simulink model "PlanarChassisVehicleModel"  (R2021a)
settings: Solver=VariableStepAuto  StartTime=0.0  StopTime=10.0  RelTol=1e-3
(part 1 of 2)
settings Model: Creator=jpchi  LastModifiedBy=jpchi

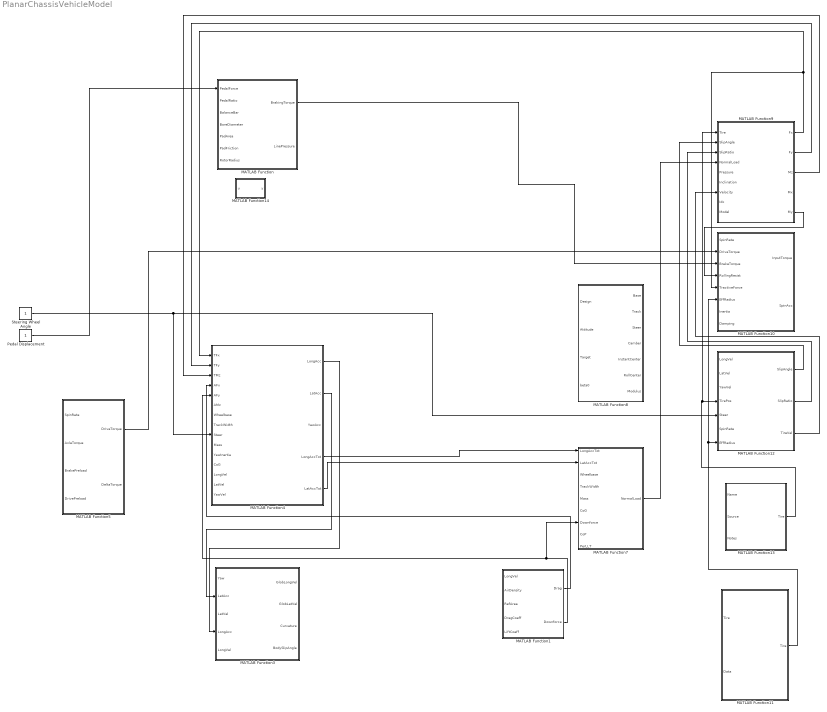
== system PlanarChassisVehicleModel ==
  MATLAB Function : MATLAB Function  TreatAsAtomicUnit=on
  MATLAB Function1 : MATLAB Function  TreatAsAtomicUnit=on
  MATLAB Function10 : MATLAB Function  TreatAsAtomicUnit=on
  MATLAB Function11 : MATLAB Function  TreatAsAtomicUnit=on
  MATLAB Function12 : MATLAB Function  TreatAsAtomicUnit=on
  MATLAB Function13 : MATLAB Function  TreatAsAtomicUnit=on
  MATLAB Function14 : MATLAB Function  TreatAsAtomicUnit=on
  MATLAB Function3 : MATLAB Function  TreatAsAtomicUnit=on
  MATLAB Function4 : MATLAB Function  TreatAsAtomicUnit=on
  MATLAB Function5 : MATLAB Function  TreatAsAtomicUnit=on
  MATLAB Function7 : MATLAB Function  TreatAsAtomicUnit=on
  MATLAB Function8 : MATLAB Function  TreatAsAtomicUnit=on
  MATLAB Function9 : MATLAB Function  TreatAsAtomicUnit=on
  Pedal Displacement : Constant
  Steering Wheel Angle : Constant
  wires:
  Pedal Displacement/1 -> MATLAB Function/1(PedalForce)
  MATLAB Function12/1(SlipAngle) -> MATLAB Function9/2(SlipAngle)
  MATLAB Function12/2(SlipRatio) -> MATLAB Function9/3(SlipRatio)
  MATLAB Function/1(BrakingTorque) -> MATLAB Function10/3(BrakeTorque)
  Steering Wheel Angle/1 -> MATLAB Function4/9(Steer), MATLAB Function12/5(Steer)
  MATLAB Function9/1(Fx) -> MATLAB Function4/1(TFx), MATLAB Function10/5(TractiveForce)
  MATLAB Function9/2(Fy) -> MATLAB Function4/2(TFy)
  MATLAB Function9/3(Mz) -> MATLAB Function4/3(TMz)
  MATLAB Function9/5(My) -> MATLAB Function10/4(RollingResist)
  MATLAB Function12/3(TireVel) -> MATLAB Function9/7(Velocity)
  MATLAB Function4/1(LongAcc) -> MATLAB Function3/4(LongAcc)
  MATLAB Function4/2(LatAcc) -> MATLAB Function3/2(LatAcc)
  MATLAB Function5/1(DriveTorque) -> MATLAB Function10/2(DriveTorque)
  MATLAB Function11/1(Tire) -> MATLAB Function12/7(EffRadius), MATLAB Function10/6(EffRadius)
  MATLAB Function13/1(Tire) -> MATLAB Function9/1(Tire), MATLAB Function12/4(TirePos)
  MATLAB Function1/1(Drag) -> MATLAB Function4/4(AFx)
  MATLAB Function1/2(Downforce) -> MATLAB Function7/7(Downforce), MATLAB Function4/5(AFy)
  MATLAB Function4/4(LongAccTot) -> MATLAB Function7/1(LongAccTot)
  MATLAB Function4/5(LatAccTot) -> MATLAB Function7/2(LatAccTot)
  MATLAB Function7/1(NormalLoad) -> MATLAB Function9/4(NormalLoad)

== matlab function PlanarChassisVehicleModel/MATLAB Function7 ==
  data: LongAccTot input; NormalLoad output; LatAccTot input; Wheelbase input; TrackWidth input; Mass input; CoG input; Downforce input; CoP input; PerLLT input
function NormalLoad  = SimplifiedWeightTransfer( LongAccTot, LatAccTot, ...
        Wheelbase, TrackWidth, Mass, CoG, Downforce, CoP, PerLLT ) 
%% SimplifiedWeightTransfer - Simplified Normal Loads
% Computes tire normal loads using simplified weight transfer and
% aerodynamic loading.
% 
% Inputs:
%   LongAccTot - (n,1 numeric) Total Longitudinal Acceleration     {a_x}   [m/s^2]
%   LatAccTot  - (n,1 numeric) Total Lateral Acceleration          {a_y}   [m/s^2]
%   Wheelbase  - (n,1 numeric) Wheelbase                           {L}     [m]
%   TrackWidth - (n,2 numeric) Track Width                         {t_w}   [m]
%   Mass       - (n,1 numeric) Total Vehicle Mass                  {m}     [kg]
%   CoG        - (n,3 numeric) Center of Gravity                   {CoG}   [m]
%   Downforce  - (n,1 numeric) Aerodynamic Downforce               {A_F_z} [N]
%   CoP        - (n,3 numeric) Center of Pressure                  {CoP}   [m]
%   PerLLT     - (n,1 numeric) Percent Front Lateral Load Transfer {%_LLT} [ ]
%
% Outputs:
%   NormalLoad - (n,4 numeric) Tire Normal Loads                   {T_F_z} [N]
%
% Notes:
%
% Author(s): 
% Blake Christierson (bechristierson@ucdavis.edu) [Sep 2018 - Jun 2021] 
% 
% Last Updated: 30-May-2021

%% Test Case
if nargin == 0
    LongAccTot = -0.5 .* 9.81;
    LatAccTot  =  0.7 .* 9.81;
    
    Wheelbase = 1.575;
    TrackWidth = [1.22, 1.23];
    
    Mass = 275;
    CoG  = [(0.47-0.5)*Wheelbase, 0, 0.25];
    
    Downforce = 200;
    CoP  = [(0.4-0.5)*Wheelbase, 0, 0];
    
    PerLLT = 0.6;
    
    [NormalLoad] = SimplifiedWeightTransfer( LongAccTot, LatAccTot, ...
        Wheelbase, TrackWidth, Mass, CoG, Downforce, CoP, PerLLT ) %#ok<NOPRT>
    
    return
end

%% Computation
NormalLoad = zeros( [size( LongAccTot ), 4] );

%%% Total Weight Transfer
dFzx = Mass .* LongAccTot .* CoG(:,3) ./ Wheelbase;
dFzy = Mass .* LatAccTot  .* CoG(:,3) ./ mean(TrackWidth, 2);

%%% Static Wheel Loads
MassBal = (CoG(:,1) + Wheelbase./2) ./ Wheelbase;
AeroBal = (CoP(:,1) + Wheelbase./2) ./ Wheelbase;

NormalLoad(:,1:2) = (MassBal .* Mass .* 9.81 + AeroBal .* Downforce) / 2;
NormalLoad(:,3:4) = ((1-MassBal) .* Mass .* 9.81 + (1-AeroBal) .* Downforce) / 2;

%%% Dynamic Wheel Loads
NormalLoad(:,1) = NormalLoad(:,1) + (-0.5.*dFzx - PerLLT    .*dFzy)/2;
NormalLoad(:,2) = NormalLoad(:,2) + (-0.5.*dFzx + PerLLT    .*dFzy)/2;
NormalLoad(:,3) = NormalLoad(:,3) + ( 0.5.*dFzx - (1-PerLLT).*dFzy)/2;
NormalLoad(:,4) = NormalLoad(:,4) + ( 0.5.*dFzx + (1-PerLLT).*dFzy)/2;

end

== matlab function PlanarChassisVehicleModel/MATLAB Function8 ==
  data: Design input; Base output; Attitude input; Target input; beta0 input; Track output; Steer output; Camber output; InstantCenter output; RollCenter output; Modulus output
function [Base, Track, Steer, Camber, InstantCenter, RollCenter, Modulus] = ...
    KinematicsEvaluation( Design, Attitude, Target, beta0 )
%% Define Coordinate Transformations
if strcmp(Target.Axle, 'Front')
    L = Target.Wheelbase;
else
    L = -Target.Wheelbase;
end

RotX = @(t) [1       0       0      ;  0       cosd(t) sind(t);  0       -sind(t) cosd(t)];
RotY = @(t) [cosd(t) 0       sind(t);  0       1       0      ; -sind(t)  0       cosd(t)];
RotZ = @(t) [cosd(t) sind(t) 0      ; -sind(t) cosd(t) 0      ;  0        0       1      ];

% bTw = @(pW,phi,theta) RotX(phi)    * RotY(theta) * (pW - Target.CG' - [L/2 0 0]'); %world to body
wTb = @(pB,phi,theta) RotY(theta)' * RotX(phi)'  *  pB + Target.CG' + [-L/2 0 Attitude.Ride-50.8]'; %body to world


% tTw = @(pW,xT,yT,gamma,phi,delta) RotZ(delta) * RotX(gamma)  * RotY(phi) * (pW - [xT yT Target.Rl]'); %world to tire
% wTt = @(pT,xT,yT,gamma,phi,delta) RotY(phi)'  * RotX(gamma)' * RotZ(delta)' *  pT + [xT yT Target.Rl]' ; %old copy - tire to world
% wTt = @(pT,xT,yT,gamma,delta) RotX(gamma)' * RotZ(delta)' *  pT + [xT yT 0]' ; %tire to world
    
% bTw = @(pW,phi,theta) RotX(phi)    * RotY(theta) * (pW - Target.CG' - [L/2 0 0]');
wTb = @(pB,phi,theta) RotY(theta)' * RotX(phi)'  *  pB + Target.CG' + [-L/2 0 Attitude.Ride-50.8]';

%tTw = @(pW,xT,yT,gamma,phi,delta) RotZ(delta) * RotX(gamma)  * RotY(phi) * (pW - [xT yT Target.Rl]');
% wTt = @(pT,xT,yT,gamma,phi,delta) RotY(phi)'  * RotX(gamma)' * RotZ(delta)' *  pT + [xT yT Target.Rl]' ;

% whTt = @
tTwh = @(pWH,camber,KPI,caster) RotY(caster)' * RotX(KPI)' * ( ( RotX(-camber)' * pWH ) + [0 Target.Scrub 0]' ) + [0 0 Target.Rl/cosd(KPI)]';
% tbTwh = @ (pWH) pWH - Design.tr;

% laTb = @(pB,beta) RotX(beta)            * RotZ(Design.a.LA(2))  * RotY(Design.a.LA(1)) * (pB - (Design.p.LAb + [L/2 0 Target.Ride-Target.CG(3)]')); %body to lower a-arm
bTla = @(pA,beta) RotY(Design.a.LA(1))' * RotZ(Design.a.LA(2))' * RotX(beta)'          *  pA +  Design.p.LAb + [L/2 0 Target.Ride-Target.CG(3)]'  ; %lower a-arm to body

% uaTb = @(pB,beta) RotX(beta)            * RotZ(Design.a.UA(2))  * RotY(Design.a.UA(1)) * (pB - (Design.p.UAb + [L/2 0 Target.Ride-Target.CG(3)]')); %body to upper a-arm
bTua = @(pA,beta) RotY(Design.a.UA(1))' * RotZ(Design.a.UA(2))' * RotX(beta)'          *  pA +  Design.p.UAb + [L/2 0 Target.Ride-Target.CG(3)]'  ; %upper a-arm to body

% lbTla = @(pA ,beta1,beta2,beta3) RotZ(beta3)  * RotX(beta1)  * RotY(beta2)  * (pA  - [0 Design.L.LA 0]'); %lower a-arm to lower ball joint
laTlb = @(pLB,beta1,beta2,beta3) RotY(beta2)' * RotX(beta1)' * RotZ(beta3)' *  pLB + [0 Design.L.LA 0]' ; %lower ball joint to lower a-arm

lbTt = @(pT ) pT  - Design.p.LBt; %tire to lower ball joint
% tTlb = @(pLB) pLB + Design.p.LBt; %lower ball joint to tire

% trTb = @(pB ,beta1,beta2) RotZ(beta2)  * RotX(beta1)  * (pB  - (Design.p.TAb + [L/2 Attitude.Steer Target.Ride-Target.CG(3)]')); %body to tie rod
bTtr = @(pTR,beta1,beta2) RotX(beta1)' * RotZ(beta2)' *  pTR +  Design.p.TAb + [L/2 Attitude.Steer Target.Ride-Target.CG(3)]'  ; %tie rod to body

% laTb = @(pB,beta) RotX(beta)            * RotZ(Design.a.LA(2))  * RotY(Design.a.LA(1)) * (pB - (Design.p.LAb + [L/2 0 Target.Ride-Target.CG(3)]'));
bTla = @(pA,beta) RotY(Design.a.LA(1))' * RotZ(Design.a.LA(2))' * RotX(beta)'          *  pA +  Design.p.LAb + [L/2 0 Target.Ride-Target.CG(3)]'  ; 

% uaTb = @(pB,beta) RotX(beta)            * RotZ(Design.a.UA(2))  * RotY(Design.a.UA(1)) * (pB - (Design.p.UAb + [L/2 0 Target.Ride-Target.CG(3)]')); 
bTua = @(pA,beta) RotY(Design.a.UA(1))' * RotZ(Design.a.UA(2))' * RotX(beta)'          *  pA +  Design.p.UAb + [L/2 0 Target.Ride-Target.CG(3)]'  ;

% lbTla = @(pA ,beta1,beta2,beta3) RotZ(beta3)  * RotX(beta1)  * RotY(beta2)  * (pA  - [0 Design.L.LA 0]'); 
laTlb = @(pLB,beta1,beta2,beta3) RotY(beta2)' * RotX(beta1)' * RotZ(beta3)' *  pLB + [0 Design.L.LA 0]' ; 

lbTt = @(pT ) pT  - Design.p.LBt; 
% tTlb = @(pLB) pLB + Design.p.LBt; 

% trTb = @(pB ,beta1,beta2) RotZ(beta2)  * RotX(beta1)  * (pB  - (Design.p.TAb + [L/2 Attitude.Steer Target.Ride-Target.CG(3)]')); 
bTtr = @(pTR,beta1,beta2) RotX(beta1)' * RotZ(beta2)' *  pTR +  Design.p.TAb + [L/2 Attitude.Steer Target.Ride-Target.CG(3)]'  ;

%% Optimization Problem Setup & Execution
if nargin < 4
    beta0 = [ 1, ... % Lower A-Arm Rotation
              5, ... % Upper A-Arm Rotation
              0, 0, ... % Tie Rod (x,z)-Axis Rotations
              0, 0, 0]; % Lower Ball Joint (x,y,z)-Axis Rotations
end

lb = [-10 -20 -20 -30 -10 -10 -40];
ub = [ 30  35  30  30  10  10  40];

ObjFun = @(beta) ObjectiveFunction( beta, Design, Attitude, Target );
[beta, fval] = fmincon( ObjFun, beta0, [], [], [], [], lb, ub, [], optimset( 'Display', 'off' ) );

[Base, Track, Steer, Camber, InstantCenter, RollCenter, Modulus] = ...
    SuspensionMetrics( beta, Attitude, Target );

%%% Local Functions
    function Fval = ObjectiveFunction( beta, Design, Attitude, Target )
        UB = bTla( laTlb( lbTt(Design.p.UBt), beta(5), beta(6), beta(7) ), beta(1) ) - ...
             bTua( [0 Design.L.UA 0]', beta(2) );
        
        TB = bTla( laTlb( lbTt(Design.p.TBt), beta(5), beta(6), beta(7) ), beta(1) ) - ...
             bTtr( [0 Design.L.TR 0]', beta(3), beta(4) );
        
        oT = wTb( bTla( laTlb( -Design.p.LBt, beta(5), beta(6), beta(7) ), beta(1) ), Attitude.Roll, Attitude.Pitch );
         
        Rl = oT(3) - Target.Rl;
        
        Fval = norm(UB) + norm(TB) + Rl.^2;
    end

    function [Base, Track, Steer, Camber, InstantCenter, RollCenter, Modulus] = ...
            SuspensionMetrics( beta, Attitude, Target )       
        %%% Wheel Position & Orientation
        % Wheel Position
        T = wTb( bTla( laTlb( lbTt([0 0 0]'), beta(5), beta(6), beta(7) ), beta(1) ), Attitude.Roll, Attitude.Pitch );
        % T = wTt([0 0 0]', Steer, Camber)
        Base = T(1);
        Track = T(2);
         
        % Solve for Tire Unit Vectors
        xT = wTb( bTla( laTlb( lbTt([1 0 0]'), beta(5), beta(6), beta(7) ), beta(1) ), Attitude.Roll, Attitude.Pitch );
        % xT = wTt([1 0 0]', Steer, Camber)
        yT = wTb( bTla( laTlb( lbTt([0 1 0]'), beta(5), beta(6), beta(7) ), beta(1) ), Attitude.Roll, Attitude.Pitch );
        % yT = wTt([0 1 0]', Steer, Camber)
        zT = wTb( bTla( laTlb( lbTt([0 0 1]'), beta(5), beta(6), beta(7) ), beta(1) ), Attitude.Roll, Attitude.Pitch );
        % zT = wTt([0 0 1]', Steer, Camber)
        
        xT = xT - T;
        yT = yT - T;
        zT = zT - T;
         
        % Solve for Tire Positions
        posT = wTb( bTla( laTlb( lbTt( tTwh([0 0 0]', Target.Camber, Target.KPI, Target.Caster) ), beta(5), beta(6), beta(7) ),...
            beta(1) ), Attitude.Roll, Attitude.Pitch );
        
        % Solve for Steer & Camber [Sign Issues]
        Camber = acosd( dot( yT, [0 0 1]' ) ) - 90; % Camber Angle [deg]

        k = cross( zT, [0 0 1]' ) ./ sind(Camber); % Camber Rotation Vector
        
        yTa = yT*cosd(Camber) + cross(k,yT)*sind(Camber) + ...
            k*dot(k,yT)*(1-cosd(Camber)); % Ground Parallel Longitudinal Tire Axis
        yTa = yTa ./ norm(yTa);
        
        Steer = -sign(yTa(1)) * acosd( dot( yTa, [0 1 0]' ) ); % Steer Angle [deg]
        
        %%% Roll Geometry Metrics
        pLA = wTb( bTla( [0 0 0]', beta(1) ), Attitude.Roll, Attitude.Pitch );
        pUA = wTb( bTua( [0 0 0]', beta(2) ), Attitude.Roll, Attitude.Pitch );
        pTA = wTb( bTtr( [0 0 0]', beta(3), beta(4) ), Attitude.Roll, Attitude.Pitch );
        
        pLB = wTb( bTla( [0 Design.L.LA 0]', beta(1) ), Attitude.Roll, Attitude.Pitch );
        pUB = wTb( bTua( [0 Design.L.UA 0]', beta(2) ), Attitude.Roll, Attitude.Pitch );
        pTB = wTb( bTtr( [0 Design.L.TR 0]', beta(3), beta(4) ), Attitude.Roll, Attitude.Pitch );
               
        InstantCenter = LineIntersection( pLA(2:3), pLB(2:3), pUA(2:3), pUB(2:3) );
        RollCenter = LineIntersection( InstantCenter, [Track,0], [0,0], [0,1] );
        
        %%% KPI / Scrub Calculator
        
        %%% Steering Effort
%         % Solve for Tire Forces
%         Tire = Target.TireParameter.Tire.Pacejka;
%         SlipAngle   = Steer;         %[degrees]
%         SlipRatio   = 0.00;             %[ ] Assume no slip
%         NormalLoad  = 270 * 9.81/4;  %[N] About 1/4 the weight of the car
%         Pressure    = 70;            %[kPa] 10 psi
%         Inclination = Target.Camber; %[degrees]
%         Velocity    = 10;            %[m/s]
%         Idx         = 1;             %[ ]
%         Model       = struct( 'Pure', 'Pacejka', 'Combined', 'MNC' );
%         
%         [Fx, Fy, Mz, ~, ~] = ContactPatchLoads( Tire, SlipAngle, ...
%             SlipRatio, NormalLoad, Pressure, Inclination, Velocity, Idx, Model );
%         
%         % Solve for Moments from tire and tie rod
%         ToeBase = T-pTB; %distance from tie rod pickup point to center of wheel
%         disT = posT - T; %posT is contact patch, T is center of wheel
%         dirTR = ( pTB-pTA ) ./ ( norm( pTB-pTA ) ); %direction of the force in the tie rod
%         
%         %Solve for Modulus
%         TireForce = [Fx, Fy, Mz]; %tire forces matrix from tire model
%         TireDirection = [ xT; yT ]; %tire direction matrix
%         Modulus = zeros( size(TireForce) ); %initiailize modulus matrix
%         
%         for i = size(TireForce)
%             if i <= size(TireDirection,1)
%                 ModulusMoment = cross( disT, TireDirection(i,:) ); %Tire Moment
%             else
%                 ModulusMoment = [ 0, 0, 1 ]; %Tire Moment
%             end
%             Modulus(i) = [0, 0, ModulusMoment(3)] ./ (cross( ToeBase, dirTR) );
%         end
%         
%         %Solve for Steering Effort
%         TieRodForce = TireForce.*Modulus'; %Solves force into the tie rod
%         SteeringEffort = TieRodForce(2)*( 0.08788 / ( 2*pi ) ); %torque at the steering wheel needed to turn wheel [N*m] (rack travel 87.88mm/deg)
        Modulus = 0;
        
        %%% Debugging
        %{ 
        plot3( LA(1), LA(2), LA(3), 'bx', ...
               UA(1), UA(2), UA(3), 'rx', ...
               TA(1), TA(2), TA(3), 'gx', ...
               LB(1), LB(2), LB(3), 'b+', ...
               UB(1), UB(2), UB(3), 'r+', ...
               TB(1), TB(2), TB(3), 'g+', ...
                T(1),  T(2),  T(3), 'mx');
        quiver3( 0, 0, 0, yT(1), yT(2), yT(3) ); hold on;
        %}
    end

    function pX = LineIntersection(p1, p2, p3, p4)
        pX(1) = det( [det( [p1(1) p1(2); p2(1) p2(2)] ), det( [p1(1) 1; p2(1) 1] ); ...
                      det( [p3(1) p3(2); p4(1) p4(2)] ), det( [p3(1) 1; p4(1) 1] )] ) ./ ...
                det( [det( [p1(1) 1    ; p2(1) 1    ] ), det( [p1(2) 1; p2(2) 1] ); ...
                      det( [p3(1) 1    ; p4(1) 1    ] ), det( [p3(2) 1; p4(2) 1] )] ); 
                  
        pX(2) = det( [det( [p1(1) p1(2); p2(1) p2(2)] ), det( [p1(2) 1; p2(2) 1] ); ...
                      det( [p3(1) p3(2); p4(1) p4(2)] ), det( [p3(2) 1; p4(2) 1] )] ) ./ ...
                det( [det( [p1(1) 1    ; p2(1) 1    ] ), det( [p1(2) 1; p2(2) 1] ); ...
                      det( [p3(1) 1    ; p4(1) 1    ] ), det( [p3(2) 1; p4(2) 1] )] );
    end
end

== matlab function PlanarChassisVehicleModel/MATLAB Function9 ==
  data: Tire input; Fx output; SlipAngle input; SlipRatio input; NormalLoad input; Pressure input; Inclination input; Velocity input; Idx input; Model input; Fy output; Mz output; Mx output; My output
function [Fx, Fy, Mz, Mx, My] = ContactPatchLoads( Tire, ...
    SlipAngle, SlipRatio, ...
    NormalLoad, Pressure, Inclination, Velocity, ...
    Idx, Model )
%% ContactPatchLoads - Tire Load Evaluation
% This script evaluates a Pacejka contact patch tire model using the
% formatted by TireModelFittingMain(). 
% 
% Inputs:
%   Tire          - (struct)      Pacejka Parameters
%   SlipAngle     - (n,1 numeric) Slip Angle          {alpha} [deg]
%   SlipRatio     - (n,1 numeric) Slip Ratio          {kappa} [ ]
%   NormalLoad    - (n,1 numeric) Normal Load         {F_z}   [N]
%   Pressure      - (n,1 numeric) Inflation Pressure  {P_i}   [kPa]
%   Inclination   - (n,1 numeric) Inclination Angle   {gamma} [deg]
%   Velocity      - (n,1 numeric) Center Velocity     {v_c}   [m/s]
%   Idx           - (n,1 numeric) Corner Idx          {1-4}   [ ]
%   Model         - (struct)      Fidelity Choices 
%       .Pure     - (char)        Pure Slip Model     {'Linear', 'Pacejka'}
%       .Combined - (char)        Combined Slip Model {'Pure', 'MNC', 'Pacejka'}
%
% Outputs:
%   Fx - (n,1 numeric) Longitudinal (Tractive) Force {F_x} [N]
%   Fy - (n,1 numeric) Lateral Force                 {F_y} [N]
%   Mz - (n,1 numeric) Aligning Moment               {M_z} [N-m]
%   Mx - (n,1 numeric) Overturning Moment            {M_x} [N-m]
%   My - (n,1 numeric) Rolling Resistance            {M_y} [N-m]
%
% Notes:
%   Pacejka combined slip model is not currently implemented (4/2/21) and
%   when the model does become available the model compatibility checks
%   should be reformatted.
%
% Author(s): 
% Blake Christierson (bechristierson@ucdavis.edu) [Sep 2018 - Jun 2021] 
% Carlos Lopez       (calopez@ucdavis.edu       ) [Jan 2019 -         ]
% Leonardo Howard    (leohoward@ucdavis.edu     ) [Jan 2021 -         ]
% Tristan Pham       (atlpham@ucdavis.edu       ) [Jan 2021 -         ]
% 
% Last Updated: 23-Oct-2021

%% Test Case
if nargin == 0
    warning('Executing SlipEstimation() Test Case')
    
    addpath( genpath( fileparts( which( 'ContactPatchLoads.m' ) ) ) );
    load('Models\TestTire.mat'); %#ok<LOAD>
    
    %%% Nominal Test Case Conditions
    Pressure    = 70;
    Inclination = 1;
    Velocity    = 10;
    Idx         = 1;
    Model       = struct( 'Pure', 'Pacejka', 'Combined', 'MNC' );
    
    %%% Slip-Load Plots 
    SlipRatio = linspace(- 1, 1,51);
    SlipAngle = linspace(-20,20,51);
    
    NormalLoad  = 0:100:2000;
        
    [~         , SlipRatio] = meshgrid( NormalLoad, SlipRatio );
    [NormalLoad, SlipAngle] = meshgrid( NormalLoad, SlipAngle );
    
    [Fx, Fy, Mz, Mx, My] = ContactPatchLoads( Tire, ...
        SlipAngle, SlipRatio, ...
        NormalLoad, Pressure, Inclination, Velocity, ...
        Idx, Model );
     
    figure
    sgtitle( {'Slip-Load Surfaces', ...
        ['$P_{i} ='  , num2str(Pressure)   , '$ [$kPa$],' ...
          '$\gamma = ', num2str(Inclination), '$ [$deg$]']} )
      
    subplot(3,2,1)
    surf( SlipRatio, NormalLoad, Fx )
    xlabel( '$\kappa$ [ ]' )
    ylabel( '$F_{z}$ [$N$]' )
    zlabel( '$F_{x}$ [$N$]' )
    title( 'Longitudinal Force' )
    
    subplot(3,2,2)
    surf( SlipAngle, NormalLoad, Fy )
    xlabel( '$\alpha$ [$deg$]' )
    ylabel( '$F_{z}$ [$N$]' )
    zlabel( '$F_{y}$ [$N$]' )
    title( 'Lateral Force' )
    
    subplot(3,2,3)
    surf( SlipAngle, NormalLoad, Mz )
    xlabel( '$\alpha$ [$deg$]' )
    ylabel( '$F_{z}$ [$N$]' )
    zlabel( '$M_{z}$ [$Nm$]' )
    title( 'Aligning Moment' )
    
    subplot(3,2,4)
    surf( SlipAngle, NormalLoad, Mx )
    xlabel( '$\alpha$ [$deg$]' )
    ylabel( '$F_{z}$ [$N$]' )
    zlabel( '$M_{x}$ [$Nm$]' )
    title( 'Overturning Moment' )
    
    subplot(3,2,5)
    surf( SlipRatio, NormalLoad, My )
    xlabel( '$\kappa$ [ ]' )
    ylabel( '$F_{z}$ [$N$]' )
    zlabel( '$M_{y}$ [$Nm$]' )
    title( 'Rolling Resistance' )
      
    %%% Friction Ellipse Plotting
    SlipRatio = linspace(- 1, 1,51);
    SlipAngle = linspace(-20,20,51);
    
    [SlipRatio, SlipAngle] = meshgrid( SlipRatio, SlipAngle );
    
    NormalLoad = 700;
    
    [Fx, Fy, ~, ~, ~] = ContactPatchLoads( Tire, ...
        SlipAngle, SlipRatio, ...
        NormalLoad, Pressure, Inclination, Velocity, ...
        Idx, Model );

    ColorMap = colormap( 'parula' );
    figure
    for i = 1 : size( SlipAngle, 1)
        plot( Fy(i,:), Fx(i,:), 'Color', ...
            ColorMap( round( (SlipAngle(i,1)-SlipAngle(1)) .* ...
                (length(ColorMap)-1) ./ diff( SlipAngle([1 end]) )) + 1, : ) ); hold on;
    end
    
    for j = 1 : size( SlipRatio, 2)
        plot( Fy(:,j), Fx(:,j), 'Color', ...
            ColorMap( round( (SlipRatio(1,j)-SlipRatio(1)) .* ...
                (length(ColorMap)-1) ./ diff( SlipRatio([1 end]) )) + 1, : ) );
    end
    
    xlabel( 'Lateral Force, $F_{y}$ [$N$]' ); 
    ylabel( 'Longitudinal Force, $F_{x}$ [$N$]' );
    title( 'Friction Ellipse' )
    
    %%% Inclination Sensitivity
    Inclination = -3:0.05:3;
    
    SlipRatio = linspace(- 1, 1,51);
    SlipAngle = linspace(-20,20,51);
    
    [~          , SlipRatio] = meshgrid( Inclination, SlipRatio );
    [Inclination, SlipAngle] = meshgrid( Inclination, SlipAngle );
    
    [Fx, Fy, ~, ~, ~] = ContactPatchLoads( Tire, ...
        SlipAngle, SlipRatio, ...
        NormalLoad, Pressure, Inclination, Velocity, ...
        Idx, Model );
    
    figure
    plot( Inclination(1,:), max(abs(Fx),[],1)./max(abs(Fx),[],'all') ); hold on;
    plot( Inclination(1,:), max(abs(Fy),[],1)./max(abs(Fy),[],'all') )
    
    xlabel( 'Inclination, $\gamma$ [$deg$]' )
    ylabel( 'Normalized Grip' )
    title( 'Inclination Sensitivity')
    legend( '$F_{x}$', '$F_{y}$' )
    
    %%% Single Evaluation
    Inclination = 1;
    SlipAngle = 5;
    SlipRatio = 0.03;
    
    [Fx, Fy, Mz, Mx, My] = ContactPatchLoads( Tire, ...
        SlipAngle, SlipRatio, ...
        NormalLoad, Pressure, Inclination, Velocity, ...
        Idx, Model );
    
    return;
end

%% Model Compatibility Check
if ~ismember(Model.Pure, {'Linear', 'Pacejka'})
    error('Please choose either ''Linear'' or ''Pacejka'' for the pure slip model')
elseif ~ismember(Model.Combined, {'Pure', 'MNC'})
    if strcmp(Model.Combined, 'Pacejka')
        error('The Pacejka combined slip model is not implemented (4/2/21)')
    else
        error('Please choose either ''Pure'' or ''MNC'' for the combined slip model')
    end
end

%% Main Evaluation
%%% Slip Angle Conversion
SlipAngle = deg2rad(SlipAngle);

%%% Left-Right Side Orientation Manipulation
% Ensures model conicity & ply-steer are symmetric to prevent drift
SlipAngle = SlipAngle .* (-1).^(mod(Idx+1,2));
Inclination   = Inclination   .* (-1).^(mod(Idx+1,2));

%%% Nondimensional Load & Pressure
dFz = (NormalLoad - Tire.Pacejka.Fzo) ./ Tire.Pacejka.Fzo;
dPi = (Pressure - Tire.Pacejka.Pio) ./ Tire.Pacejka.Pio;

%%% Evaluate Pure Slip Forces & Aligning Moment
[Fx0, Kxk, Kappa0] = EvaluateFx0( Tire, SlipAngle, SlipRatio, ...
    NormalLoad, dFz, Pressure, dPi, Inclination, Velocity, Idx, Model ); 

[Fy0, By, Cy, Kya, Hy, Vy, Alpha0] = EvaluateFy0( Tire, SlipAngle, SlipRatio, ...
    NormalLoad, dFz, Pressure, dPi, Inclination, Velocity, Idx, Model ); 
    
[Fyo, ~, ~, ~, ~, ~, Alphao] = EvaluateFy0( Tire, SlipAngle, SlipRatio, ...
    NormalLoad, dFz, Pressure, dPi, 0  , Velocity, Idx, Model );

[Mz0, Bt, Ct, Dt, Et, Ht, Br, Cr, Dr, Hf] = EvaluateMz0( Tire, SlipAngle, SlipRatio, ...
    NormalLoad, dFz, Pressure, dPi, Inclination, Velocity, Idx, Model, ...
    Fyo, By, Cy, Kya, Hy, Vy );

%%% Combined Slip Force Models 
switch Model.Combined
    case 'Pure' % Pure Slip Only Model
        Fx  = Fx0;
        Fy  = Fy0;   

    case 'MNC' % Modified-Nicolas-Comstock Combined Slip Model
        [Fx, Fy ]  = MNCCombinedSlipForces( Tire, ...
            SlipAngle, SlipRatio, Fx0, Fy0, Kxk, Kya, Kappa0, Alpha0 );
        [~ , Fyp]  = MNCCombinedSlipForces( Tire, ...
            SlipAngle, SlipRatio, Fx0, Fyo, Kxk, Kya, Kappa0, Alphao );

    case 'MF6_1' % Combined Slip Pacejka MF6.1 Model
        % Not Implemented
end

%%% Evaluate Combined Slip Aligning Moment (Mz)
if strcmpi( Model.Combined, 'Pure' )
    Mz = Mz0;
else
    Mz = EvaluateMz( Tire, SlipAngle, SlipRatio, ...
        NormalLoad, dFz, Pressure, dPi, Inclination, Velocity, Idx, Model, ...
        Fx, Fy, Fyp, Kxk, Kya, Bt, Ct, Dt, Et, Ht, Br, Cr, Dr, Hf );
end

%%% Evaluate Moment & Rolling Resistance
Mx = EvaluateMx( Tire, SlipAngle, SlipRatio, ...
    NormalLoad, dFz, Pressure, dPi, Inclination, Velocity, Idx, Model, Fy );

My = EvaluateMy( Tire, SlipAngle, SlipRatio, ...
    NormalLoad, dFz, Pressure, dPi, Inclination, Velocity, Idx, Model, Fx );

%%% Pure Slip Longitudinal Force Evaluation (Fx0)
function [Fx0, Kxk, Kappa0] = ...
        EvaluateFx0( Tire, ~, Kappa, Fz, dFz, ~, dPi, Inc, ~, ~, Model )
    
    % Evaluate P6 Pacejka
    Cx = Tire.Pacejka.p.C.x(1) .* Tire.Pacejka.L.C.x;

    Dx = (Tire.Pacejka.p.D.x(1) + Tire.Pacejka.p.D.x(2).*dFz) .* ...
         (1 + Tire.Pacejka.p.P.x(3).*dPi + Tire.Pacejka.p.P.x(4).*dPi.^2) .* ...
         (1 - Tire.Pacejka.p.D.x(3).*Inc.^2).*Fz .* Tire.Pacejka.L.mu.x;

    Ex = ( Tire.Pacejka.p.E.x(1) + Tire.Pacejka.p.E.x(2).*dFz ...
        + Tire.Pacejka.p.E.x(3).*dFz.^2 ) .* ( 1 - Tire.Pacejka.p.E.x(4).*sign(Kappa) ) .* ...
        Tire.Pacejka.L.E.x;

    Kxk = Fz.*(Tire.Pacejka.p.K.x(1) + Tire.Pacejka.p.K.x(2).*dFz ) .* ...
        exp( Tire.Pacejka.p.K.x(3) .* dFz ) .* ...
        (1 + Tire.Pacejka.p.P.x(1).*dPi + Tire.Pacejka.p.P.x(2).*dPi.^2) .* ...
        Tire.Pacejka.L.K.x.k;

    Bx = Kxk ./ ( Cx.*Dx );

    Vx = Fz.*(Tire.Pacejka.p.V.x(1) + Tire.Pacejka.p.V.x(2).*dFz ) .* ...
        Tire.Pacejka.L.V.x;

    Hx = (Tire.Pacejka.p.H.x(1) + Tire.Pacejka.p.H.x(2).*dFz) .* ...
        Tire.Pacejka.L.H.x;

    % Evaluate Longitudinal Force​
    switch Model.Pure
        case 'Linear'
            Fx0 = Kxk .* Kappa;
        case 'Pacejka'
            Fx0 = Dx .* sin( Cx .* atan( (1-Ex) .* Bx.*(Kappa + Hx) + ...
                Ex.*atan( Bx.*(Kappa + Hx) ) ) ) + Vx;
    end

    % Evaluate Null Slip Ratio
    if strcmpi( Model.Combined, 'MNC' )
        Kappa0 = -Vx ./ Kxk - Hx;
        Kappa0(isnan(Kappa0)) = 0; % Can use smoothing in future
    else
        Kappa0 = [];
    end
end

%%% Pure Slip Lateral Force Evaluation (Fy0)
function [Fy0, By, Cy, Kya, Hy, Vy, Alpha0] = ...
        EvaluateFy0( Tire, Alpha, ~, Fz, dFz, ~, dPi, Inc, ~, i, Model )            
    
    % Evaluate P6 Pacejka
    Cy = Tire.Pacejka.p.C.y(1);

    Dy = (Tire.Pacejka.p.D.y(1) + Tire.Pacejka.p.D.y(2).*dFz) .* ...
         (1 + Tire.Pacejka.p.P.y(3).*dPi + Tire.Pacejka.p.P.y(4).*dPi.^2) .* ...
         (1 - Tire.Pacejka.p.D.y(3).*Inc.^2).*Fz;

    Kya = Tire.Pacejka.p.K.y(1) .* Tire.Pacejka.Fzo .* ( 1 + Tire.Pacejka.p.P.y(1).*dPi ) .* ...
        ( 1 - Tire.Pacejka.p.K.y(3).*abs(Inc) ) .* sin( Tire.Pacejka.p.K.y(4) .* ...
        atan( (Fz./Tire.Pacejka.Fzo) ./ ...
        ( ( Tire.Pacejka.p.K.y(2) + Tire.Pacejka.p.K.y(5).*Inc.^2 ) .* ...
        ( 1 + Tire.Pacejka.p.P.y(2).*dPi ) ) ) );

    Kyg0 = Fz.*(Tire.Pacejka.p.K.y(6) + Tire.Pacejka.p.K.y(7).*dFz ) .* ...
        (1 + Tire.Pacejka.p.P.y(5).*dPi );

    By = Kya ./ ( Cy.*Dy );

    Vyg = Fz.*(Tire.Pacejka.p.V.y(3) + Tire.Pacejka.p.V.y(4).*dFz ).*Inc;

    Vy = Fz.*(Tire.Pacejka.p.V.y(1) + Tire.Pacejka.p.V.y(2).*dFz ) + Vyg;

    Hy = (Tire.Pacejka.p.H.y(1) + Tire.Pacejka.p.H.y(2).*dFz ) .* (Kyg0.*Inc - Vyg ) ./ Kya;

    Ey = ( Tire.Pacejka.p.E.y(1) + Tire.Pacejka.p.E.y(2).*dFz ) .* ...
        ( 1 + Tire.Pacejka.p.E.y(5).*Inc.^2 - ...
        ( Tire.Pacejka.p.E.y(3) + Tire.Pacejka.p.E.y(4).*Inc ).*sign(Alpha + Hy) );

    % Evaluate Lateral Force
    switch Model.Pure
        case 'Linear'
            Fy0 = Kya .* Alpha;
        case 'Pacejka'
            Fy0 = (Dy .* sin( Cy .* atan( (1-Ey) .* By.*( Alpha + Hy ) + ...
                Ey .* atan( By.*( Alpha + Hy ) ) ) ) + Vy) .* (-1).^(mod(i+1,2));
    end

    % Evaluate Null Slip Angle
    if strcmpi( Model.Combined, 'MNC' )
        Alpha0 = -Vy ./ Kya - Hy;
        Alpha0(isnan(Alpha0)) = 0;
    else
        Alpha0 = [];
    end
end

%%% Evaluate Pure Slip Aligning Moment (Mz0)
function [Mz0, Bt, Ct, Dt, Et, Ht, Br, Cr, Dr, Hf] = ...
        EvaluateMz0( Tire, Alpha, ~, Fz, dFz, ~, dPi, Inc, ~, i, ~, ...
            Fyo, By, Cy, Kya, Hy, Vy )
    
    % Evaluate P6 Pacejka
    Bt = (Tire.Pacejka.q.B.z(1) + Tire.Pacejka.q.B.z(2).*dFz + ...
        Tire.Pacejka.q.B.z(3).*dFz.^2) .* ...
        (1 + Tire.Pacejka.q.B.z(5).*abs(Inc) + ...
        Tire.Pacejka.q.B.z(6).*Inc.^2);

    Ct = Tire.Pacejka.q.C.z(1);

    Dt = (Tire.Pacejka.Ro ./ Tire.Pacejka.Fzo) .* ...
        ( Tire.Pacejka.q.D.z(5) .* (Tire.Pacejka.Fzo ./ Tire.Pacejka.Ro) + ...
        Tire.Pacejka.q.D.z(1).*Fz + Tire.Pacejka.q.D.z(2).*Fz.*dFz ) .* ...
        ( 1 - Tire.Pacejka.p.P.z(1).*dPi ) .* ...
        ( 1 + Tire.Pacejka.q.D.z(3).*abs(Inc) + ...
        Tire.Pacejka.q.D.z(4).*Inc.^2 );

    Ht = Tire.Pacejka.q.H.z(1) + ...
        Tire.Pacejka.q.H.z(2).*dFz + (Tire.Pacejka.q.H.z(3) + ...
        Tire.Pacejka.q.H.z(4).*dFz).*Inc;

    Et = (Tire.Pacejka.q.E.z(1) + Tire.Pacejka.q.E.z(2).*dFz + ...
        Tire.Pacejka.q.E.z(3).*dFz.^2) .* ...
        (1 + (Tire.Pacejka.q.E.z(4) + Tire.Pacejka.q.E.z(5).*Inc).*(2/pi).* ...
        atan( Bt .* Ct .* (Alpha+Ht) ) );

    Br = Tire.Pacejka.q.B.z(10) .* By .* Cy;

    Cr = 1;

    Dr = Tire.Pacejka.Ro .* Fz .* ( ( Tire.Pacejka.q.D.z(6) + ...
        Tire.Pacejka.q.D.z(7).*dFz ) + ...
        ( ( Tire.Pacejka.q.D.z(8) + Tire.Pacejka.q.D.z(9).*dFz ) .* ...
        ( 1 + Tire.Pacejka.p.P.z(2).*dPi ) + ...
        ( Tire.Pacejka.q.D.z(10) + Tire.Pacejka.q.D.z(11).*dFz ) .* ...
        abs(Inc) ).*Inc ) .* cos( Alpha );

    Hf = Hy + Vy ./ Kya;

    % Evaluate Trail Function
    t0 = Dt.*cos( Ct.*atan( (1-Et).*(Bt.*(Alpha + Ht)) + ...
        Et.*atan( Bt.*(Alpha + Ht) ) ) ) .* cos( Alpha ) ;

    % Evaluate Residual Aligning Moment
    Mzro = Dr .* cos( Cr.*atan( Br.*(Alpha + Hf) ) ).* cos( Alpha );

    % Evaluate Pure Slip Aligning Moment (Mz0)
    Mz0 = (-t0 .* Fyo .* (-1).^(mod(i+1,2)) + Mzro) .* (-1).^(mod(i+1,2));
end

%%% Modified-Nicolas Comstock Combined Slip Forces
function [Fx, Fy] = MNCCombinedSlipForces( ~, Alpha, Kappa, Fx0, Fy0, Kxk, Kya, Kappa0, Alpha0 )
    Fx = abs(Fx0 .* Fy0 ./ sqrt( (Kappa - Kappa0).^2 .* Fy0.^2 + Fx0.^2 .* tan(Alpha - Alpha0).^2 ) .* ...
        sqrt( (Kappa - Kappa0).^2 .* Kya.^2 + (1 - abs(Kappa - Kappa0)).^2 .* cos(Alpha - Alpha0).^2 .* Fx0.^2 ) ./ Kya) .* sign(Fx0);

    Fy = abs( Fx0 .* Fy0 ./ sqrt( (Kappa - Kappa0).^2 .* Fy0.^2 + Fx0.^2 .* tan(Alpha - Alpha0).^2 ) .* ...
        sqrt( (1 - abs(Kappa - Kappa0)).^2 .* cos(Alpha - Alpha0).^2 .* Fy0.^2 + sin(Alpha - Alpha0).^2 .* Kxk.^2 ) ./ ...
        ( Kxk .* cos(Alpha - Alpha0)) ) .* sign(Fy0);
end

%%% Evaluate Combined Slip Aligning Moment (Mz)
function Mz = EvaluateMz( Tire, Alpha, Kappa, ~, dFz, ~, ~, Inc, ~, i, ~, ...
    Fx, Fy, Fyp, Kxk, Kya, Bt, Ct, Dt, Et, Ht, Br, Cr, Dr, Hf )
    
    % Equivalent Slips
    Alphat = (Alpha + (-1).^(mod(i+1,2)).*Ht );
    Alphar = (Alpha + (-1).^(mod(i+1,2)).*Hf );

    Alphateq = sqrt( Alphat.^2 + (Kxk./Kya).^2 .* Kappa.^2 ) .* sign( Alphat );
    Alphareq = sqrt( Alphar.^2 + (Kxk./Kya).^2 .* Kappa.^2 ) .* sign( Alphar );

    % Evaluate Trail Function
    t = Dt.*cos( Ct.*atan( (1-Et).*(Bt.*Alphateq) + ...
        Et.*atan(Bt.*Alphateq) ) ) .* cos( Alpha );

    % Evaluate Scrub Function
    s = Tire.Pacejka.Ro .* (Tire.Pacejka.s.s.z(1) + ...
        Tire.Pacejka.s.s.z(2) .* (Fy./Tire.Pacejka.Fzo) + ...
        (Tire.Pacejka.s.s.z(3) + Tire.Pacejka.s.s.z(4) .* dFz) .* Inc );

    % Evaluate Residual Aligning Moment
    Mzr = Dr .* cos( Cr.*atan( Br.*(Alphareq) ) ) .* cos( Alpha );

    % Evaluate Pure Slip Aligning Moment (Mz0)
    Mz = -t .* Fyp + Mzr + s .* Fx;
end

%%% Evaluate Overturning Moment
function Mx = EvaluateMx( Tire, ~, ~, Fz, ~, ~, dPi, Inc, ~, ~, ~, Fy )
    Mx = Tire.Pacejka.Ro .* Fz .* ( Tire.Pacejka.q.s.x(1) - ...
        Tire.Pacejka.q.s.x(2) .* Inc .* ( 1 + Tire.Pacejka.p.P.Mx(1).*dPi ) + ...
        Tire.Pacejka.q.s.x(3) .* Fy ./ Tire.Pacejka.Fzo + ...
        Tire.Pacejka.q.s.x(4) .* cos( Tire.Pacejka.q.s.x(5) .* ...
        ( atan( (Tire.Pacejka.q.s.x(6) .* Fz ./ Tire.Pacejka.Fzo) ) ).^2 ) .* ...
        sin( Tire.Pacejka.q.s.x(7) .* Inc + Tire.Pacejka.q.s.x(8) .* ...
        atan( Tire.Pacejka.q.s.x(9) .* Fy ./ Tire.Pacejka.Fzo ) ) + ...
        Tire.Pacejka.q.s.x(10) .* atan( Tire.Pacejka.q.s.x(11) .* Fz ./ Tire.Pacejka.Fzo ) .* Inc );
end

%%% Evaluate Rolling Resistance
function My = EvaluateMy( Tire, ~, Kappa, Fz, ~, Pi, ~, ~, V, ~, ~, Fx )
    Re = Tire.Radius.Effective( Kappa, Fz, Pi );
    Rl = Tire.Radius.Loaded( Fz, Pi );
    
    My = Fx .* (Re - Rl) + Fz .* Re .* ( Tire.Pacejka.q.s.y(1) + ...
        Tire.Pacejka.q.s.y(3) .* (V ./ Tire.Pacejka.Vo) + ...
        Tire.Pacejka.q.s.y(4) .* (V ./ Tire.Pacejka.Vo).^4 );
end
%%% Slip-Load Plots
[~         , SlipRatio] = meshgrid( NormalLoad, SlipRatio );
    [NormalLoad, SlipAngle] = meshgrid( NormalLoad, SlipAngle );
figure
    sgtitle( {'Slip-Load Surfaces', ...
        ['$P_{i} ='  , num2str(Pressure)   , '$ [$kPa$],' ...
          '$\gamma = ', num2str(Inclination), '$ [$deg$]']} )
    subplot(3,2,1)
    surf( SlipRatio, NormalLoad, Fx )
    xlabel( '$\kappa$ [ ]' )
    ylabel( '$F_{z}$ [$N$]' )
    zlabel( '$F_{x}$ [$N$]' )
    title( 'Longitudinal Force' )
    subplot(3,2,2)
    surf( SlipAngle, NormalLoad, Fy )
    xlabel( '$\alpha$ [$deg$]' )
    ylabel( '$F_{z}$ [$N$]' )
    zlabel( '$F_{y}$ [$N$]' )
    title( 'Lateral Force' )
    subplot(3,2,3)
    surf( SlipAngle, NormalLoad, Mz )
    xlabel( '$\alpha$ [$deg$]' )
    ylabel( '$F_{z}$ [$N$]' )
    zlabel( '$M_{z}$ [$Nm$]' )
    title( 'Aligning Moment' )
    subplot(3,2,4)
    surf( SlipAngle, NormalLoad, Mx )
    xlabel( '$\alpha$ [$deg$]' )
    ylabel( '$F_{z}$ [$N$]' )
    zlabel( '$M_{x}$ [$Nm$]' )
    title( 'Overturning Moment' )
    subplot(3,2,5)
    surf( SlipRatio, NormalLoad, My )
    xlabel( '$\kappa$ [ ]' )
    ylabel( '$F_{z}$ [$N$]' )
    zlabel( '$M_{y}$ [$Nm$]' )
    title( 'Rolling Resistance' )
%%% Friction Ellipse Plotting
ColorMap = colormap( 'parula' );
    figure
    for i = 1 : size( SlipAngle, 1)
        plot( Fy(i,:), Fx(i,:), 'Color', ...
            ColorMap( round( (SlipAngle(i,1)-SlipAngle(1)) .* ...
                (length(ColorMap)-1) ./ diff( SlipAngle([1 end]) )) + 1, : ) ); hold on;
    end
    for j = 1 : size( SlipRatio, 2)
        plot( Fy(:,j), Fx(:,j), 'Color', ...
            ColorMap( round( (SlipRatio(1,j)-SlipRatio(1)) .* ...
                (length(ColorMap)-1) ./ diff( SlipRatio([1 end]) )) + 1, : ) );
    end
    xlabel( 'Lateral Force, $F_{y}$ [$N$]' );
    ylabel( 'Longitudinal Force, $F_{x}$ [$N$]' );
    title( 'Friction Ellipse' )
%%% Inclination Sensitivity
figure
    plot( Inclination(1,:), max(abs(Fx),[],1)./max(abs(Fx),[],'all') ); hold on;
    plot( Inclination(1,:), max(abs(Fy),[],1)./max(abs(Fy),[],'all') )
    xlabel( 'Inclination, $\gamma$ [$deg$]' )
    ylabel( 'Normalized Grip' )
    title( 'Inclination Sensitivity')
    legend( '$F_{x}$', '$F_{y}$' )
end

== matlab function PlanarChassisVehicleModel/MATLAB Function10 ==
  data: SpinRate input; InputTorque output; DriveTorque input; BrakeTorque input; RollingResist input; TractiveForce input; EffRadius input; Inertia input; Damping input; SpinAcc output
function [InputTorque, SpinAcc] = WheelSpeed( SpinRate, DriveTorque, ...
    BrakeTorque, RollingResist, TractiveForce, EffRadius, Inertia, Damping )
%% WheelSpeed - Wheel Torque Balance & Spin Acceleration
% Calculates brake or drive torque required for steady state applications
% or the spin acceleration for transient applications.
% 
% Inputs:
%   SpinRate      - (n,1 numeric) Wheel Spin Rate       {omega} [rad/s]
%   DriveTorque   - (n,1 numeric) Drive Torque          {tau_D} [N-m]
%   BrakeTorque   - (n,1 numeric) Brake Torque          {tau_B} [N-m]
%   RollingResist - (n,1 numeric) Rolling Resistance    {M_y}   [N-m] 
%   TractiveForce - (n,1 numeric) Tractive Force        {F_x}   [N]
%   EffRadius     - (n,1 numeric) Tire Effective Radius {r_e}   [m]
%   Inertia       - (n,1 numeric) Spin Inertia          {I_s}   [kg-m^2]
%   Damping       - (n,1 numeric) Spin Damping          {b_s}   [N-m-s/rad]
% 
% Outputs:
%   InputTorque - (n,1 numeric) Axle Input Torque      {tau_{D|B}} [N-m]
%   SpinAcc     - (n,1 numeric) Tire Spin Acceleration {omega_dot} [rad/s^2]
%
% Notes:
%   Steady state computation will be enacted if BrakeTorque or DriveTorque
%   arguments are left empty.
%
% Author(s): 
% Blake Christierson (bechristierson@ucdavis.edu) [Sep 2018 - Jun 2021] 
% Joseph Sanchez     (jomsanchez@ucdavis.edu)     [Sep 2020 - Jun 2022]
%
% Last Updated: 01-Jun-2021

%% Test Cases
if nargin == 0
    %%% Test Inputs
    SpinRate = 20:20:100; 
    
    DriveTorque = 20*ones(size(SpinRate)); 
    BrakeTorque = 0*ones(size(SpinRate)); 
    
    RollingResist = -0.05*ones(size(SpinRate));
    
    TractiveForce = 300*ones(size(SpinRate));
    EffRadius     = 0.19*ones(size(SpinRate));
    
    Inertia = 0.148;
    Damping = 0.01;
    
    fprintf('Executing WheelSpeed() Test Cases: \n');
    
    %%% Steady State Test Cases
    [InputTorque, ~] = WheelSpeed( SpinRate, [], [], ...
        RollingResist, TractiveForce, EffRadius, Inertia, Damping );
    
    for i = 1:numel(InputTorque)
        fprintf('   Steady State Instance %i: \n', i);
        fprintf('      tau_i = %5.2f [N-m] \n', InputTorque(i));
    end
    
    %%% Transient Test Cases
    [~, SpinAcc] = WheelSpeed( SpinRate, DriveTorque, BrakeTorque, ...
        RollingResist, TractiveForce, EffRadius, Inertia, Damping );  
    
    for i = 1:numel(SpinAcc)
        fprintf('   Transient Instance %i: \n', i);
        fprintf('      omega_dot = %5.2f [rad/s^2] \n', SpinAcc(i));
    end
    
     return;   
end

%% Computation
if isempty( DriveTorque ) || isempty( BrakeTorque )
    %%% Steady State Input Torque
    InputTorque = TractiveForce.*EffRadius + Damping.*SpinRate + RollingResist;
        
    SpinAcc = NaN;
else
    %%% Transient Spin Acceleration
    SpinAcc = ( DriveTorque - BrakeTorque - RollingResist - ...
        TractiveForce.*EffRadius - Damping.*SpinRate ) ./ Inertia;
    
    InputTorque = NaN;
end

== matlab function PlanarChassisVehicleModel/MATLAB Function11 ==
  data: Tire input; Tire output; Data input
function Tire  = RadialDeflectionFitting( Tire,Data )
%% Radial Deflection Modeling - Loaded & Effective Radius Model
% This fits simple poly22 surfaces for the tire loaded and effective
% radius. Cornering data is used for determining loaded radius while drive,
% brake, & combined data is used to determine effective radius. If the
% drive, brake, & combined data is from a different tire (e.g. for 16"
% tires), the effective radius fit will be scaled.
% 
% Inputs:
%   Tire - (struct) FRUCDTire Object
%   Data - (struct) Formatted Structure of Calspan TTC Data via DataImport()
% 
% Outputs:
%   Tire - (struct) FRUCDTire Object with Updated Radius Property
%
% Author(s):
% Blake Christierson (bechristierson@ucdavis.edu)
% Leonardo Howard    (leohoward@ucdavis.edu     )
% Tristan Pham       (atlpham@ucdavis.edu       )
%
% Last Updated: 23-Oct-2021

%% Loaded Radius
Form = fittype( 'p00+p10*Fz+p01*Pi+p20*Fz^2+p02*Pi^2+p11*Fz*Pi', ...
    'independent', {'Fz', 'Pi'}, 'dependent', 'Rl' );

Opts = fitoptions( 'Method', 'NonlinearLeastSquares' );
Opts.Display    = 'Off';
Opts.StartPoint = [200, 0, 0, 0, 0, 0];

Loaded(1).Load     = [Data(1).Force(3,:)   , Data(2).Force(3,:)   , Data(3).Force(3,:)   ];
Loaded(1).Pressure = [Data(1).Pressure     , Data(2).Pressure     , Data(3).Pressure     ]; 
Loaded(1).Radius   = [Data(1).Radius.Loaded, Data(2).Radius.Loaded, Data(3).Radius.Loaded] .* 10;

LoadedFit{1} = fit( [Loaded(1).Load; Loaded(1).Pressure]', Loaded(1).Radius', Form, Opts );

Tire.Radius.Loaded.Form       = formula( LoadedFit{1} );
Tire.Radius.Loaded.ArgNames   = indepnames( LoadedFit{1} );
Tire.Radius.Loaded.CoeffNames = coeffnames( LoadedFit{1} );
%% Effective Radius
Effective.Load      = [Data(4).Force(3,:)      , Data(5).Force(3,:)      , Data(6).Force(3,:)      ];
Effective.Pressure  = [Data(4).Pressure        , Data(5).Pressure        , Data(6).Pressure        ];
Effective.SlipRatio = [Data(4).Slip.Ratio      , Data(5).Slip.Ratio      , Data(6).Slip.Ratio      ];
Effective.Radius    = [Data(4).Radius.Effective, Data(5).Radius.Effective, Data(6).Radius.Effective] .* 10;

%%% Scaling Data Between Incoherent Data Sets
if ~all( strcmpi({Data(2:end).Tire}, Data(1).Tire ) )
    Loaded(2).Load     = [Data(4).Force(3,:)   , Data(5).Force(3,:)   , Data(6).Force(3,:)   ];
    Loaded(2).Pressure = [Data(4).Pressure     , Data(5).Pressure     , Data(6).Pressure     ]; 
    Loaded(2).Radius   = [Data(4).Radius.Loaded, Data(5).Radius.Loaded, Data(6).Radius.Loaded] .* 10;
    
    LoadedFit{2} = fit( [Loaded(2).Load; Loaded(2).Pressure]', Loaded(2).Radius', Form, Opts );
    Tire.Radius.Loaded = fit( [Loaded(2).Load; Loaded(2).Pressure]', Loaded(2).Radius', Form, Opts );
  
    Effective.Radius = Effective.Radius .* ...
        Tire.Radius.Loaded( Tire.Pacejka.Fzo./4, Tire.Pacejka.Pio ) ./ ...
        LoadedFit{2}( Tire.Pacejka.Fzo./4, Tire.Pacejka.Pio );
end

%%% Fit Effective Radius Surface
p000 = optimvar('p000');
p001 = optimvar('p001'); p010 = optimvar('p010'); p100 = optimvar('p100');
p011 = optimvar('p011'); p101 = optimvar('p101'); p110 = optimvar('p110');
p002 = optimvar('p002'); p020 = optimvar('p020'); p200 = optimvar('p200');

x0.p000 = 200;
x0.p001 =- 50; x0.p010 = 0; x0.p100 = 0;
x0.p011 =   0; x0.p101 = 0; x0.p110 = 0;
x0.p002 =  50; x0.p020 = 0; x0.p200 = 0;

Obj = fcn2optimexpr( @ErrorRe, p000, p001, p010, p100, p011, p101, p110, p002, p020, p200 );

[Solution, ~] = Runfmincon( Obj, x0, [], 1 );
delete( findobj( 'Type', 'figure', 'Name', 'Optimization PlotFcns' ) );

Tire.Radius.Effective = @(Kappa, Fz, Pi) Solution.p000 + ...
    Solution.p001 .* Kappa + Solution.p010 .* Fz + Solution.p100 .* Pi + ...
    Solution.p011 .* Kappa .* Fz + Solution.p101 .* Kappa .* Pi + Solution.p110 .* Fz .* Pi + ...
    Solution.p002 .* Kappa.^2 + Solution.p020 .* Fz.^2 + Solution.p200 .* Pi.^2;

%% Plotting
%%% Mesh Generation
Load      = 0:250:2000;
Pressure  = 50:10:100;
SlipRatio = linspace( -0.2, 0.2, length(Pressure) );

[~   , Pressure ] = meshgrid( Load, Pressure  );
[Load, SlipRatio] = meshgrid( Load, SlipRatio );

%%% Null Slip Ratio
NullIdx = abs(Effective.SlipRatio) < 0.005;

%%% Loaded Radius Carpet Plot (Load - Pressure)
figure( 'Name', 'Radial Deflection Models' );

subplot(2,2,[1 3])
scatter3( Loaded(1).Load, Loaded(1).Radius, Loaded(1).Pressure, [], Loaded(1).Pressure, '.', ...
    'MarkerEdgeAlpha', 0.3, 'MarkerFaceAlpha', 0.3 ); hold on;

surf( Load, Tire.Radius.Loaded( Load, Pressure ), Pressure );

xlabel( 'Normal Load, $F_{z}$ [$N$]' );
ylabel( 'Loaded Radius, $r_{l}$ [$mm$]' );
zlabel( 'Pressure, $P_{i}$ [$kPa$]' );

CB = colorbar( 'TickLabelInterpreter', 'latex' );
CB.Label.String = 'Pressure, $P_{i}$ [$kPa$]';
CB.Label.Interpreter = 'latex';

view(0,90)

%%% Effective Radius Carpet Plot (Slip Ratio - Load)
subplot(2,2,2) 
scatter3( Effective.SlipRatio, Effective.Radius, Effective.Load, [], Effective.Pressure, '.', ...
    'MarkerEdgeAlpha', 0.3, 'MarkerFaceAlpha', 0.3 ); hold on;

surf( SlipRatio, Tire.Radius.Effective( SlipRatio, Load, 70 ), Load, 70.*ones(size(Load)) );

xlabel( 'Slip Ratio, $\kappa$ [ ]' );
ylabel( 'Effective Radius, $r_{e}$ [$mm$]' );
zlabel( 'Normal Load, $F_{z}$ [$N$]' );

CB = colorbar( 'TickLabelInterpreter', 'latex' );
CB.Label.String = 'Pressure, $P_{i}$ [$kPa$]';
CB.Label.Interpreter = 'latex';

view(0,90)

%%% Effective Radius Carpet Plot (Load - Pressure)
subplot(2,2,4) 
scatter3( Effective.Load(NullIdx), Effective.Radius(NullIdx), ...
    Effective.Pressure(NullIdx), [], Effective.Pressure(NullIdx), '.', ...
    'MarkerEdgeAlpha', 0.3, 'MarkerFaceAlpha', 0.3 ); hold on;

surf( Load, Tire.Radius.Effective( 0, Load, Pressure ), Pressure );

xlabel( 'Normal Load, $F_{z}$ [$N$]' );
ylabel( 'Effective Radius, $r_{e}$ [$mm$]' );
zlabel( 'Pressure, $P_{i}$ [$kPa$]' );

CB = colorbar( 'TickLabelInterpreter', 'latex' );
CB.Label.String = 'Pressure, $P_{i}$ [$kPa$]';
CB.Label.Interpreter = 'latex';

view(0,90)

%% Local Functions
function RMSE = ErrorRe( p000, p001, p010, p100, ...
        p011, p101, p110, p002, p020, p200 )
    
    Re = p000 + p001.*Effective.SlipRatio + p010.*Effective.Load + p100.*Effective.Pressure + ...
        p011.*Effective.SlipRatio.*Effective.Load + p101.*Effective.SlipRatio.*Effective.Pressure + ...
        p110.*Effective.Load.*Effective.Pressure + ...
        p002.*Effective.SlipRatio.^2 + p020.*Effective.Load.^2 + p200.*Effective.Pressure.^2;
     
    RMSE = sqrt( mean( (Re(:) - Effective.Radius(:)).^2 ) );
end

end

== matlab function PlanarChassisVehicleModel/MATLAB Function12 ==
  data: LongVel input; SlipAngle output; LatVel input; YawVel input; TirePos input; Steer input; SpinRate input; EffRadius input; SlipRatio output; TireVel output
function [SlipAngle, SlipRatio, TireVel] = SlipEstimation( ...
    LongVel, LatVel, YawVel, TirePos, Steer, SpinRate, EffRadius)

%% SlipEstimation - Slip Angle and Slip Ratio Calculations
% Estimates tire slips and center velocity from chassis velocity and a
% handful of tire states.
% 
% Inputs:
%   LongVel   - (1,1 numeric) Longitudinal Velocity {x_dot}   [m/s]
%   LatVel    - (1,1 numeric) Lateral Velocity      {y_dot}   [m/s]
%   YawVel    - (1,1 numeric) Yaw Rate              {psi_dot} [rad/s]
%   TirePos   - (n,3 numeric) [x,y,0] Tire Position {p}       [m]
%   Steer     - (n,1 numeric) Tire Steer Angle      {delta}   [deg]
%   SpinRate  - (n,1 numeric) Tire Spin Rate        {omega}   [rad/s]
%   EffRadius - (n,1 numeric) Tire Effective Radius {r_e}     [m]
% 
% Outputs:
%   SlipAngle - (n,1 numeric) Tire Slip Angle      {alpha} [deg]
%   SlipRatio - (n,1 numeric) Tire Slip Ratio      {kappa} [ ]
%   TireVel   - (n,1 numeric) Tire Center Velocity {v_c}   [m/s]
%
% Notes:
%   Typically n=4; however, may be vectorized by stacking rows.
%
% Author(s): 
% Blake Christierson (bechristierson@ucdavis.edu) [Sep 2018 - Jun 2021] 
%
% Last Updated: 1-Apr-2021

%% Test Cases
if nargin == 0
    LongVel = 10;
    LatVel = 2;
    YawVel = 0.1;
    TirePos = [ 0.84  0.66 0; ...
                0.84 -0.66 0; ...
               -0.67  0.66 0; ...
               -0.67 -0.66 0];
    
    Steer = [25; 20; -0.5; 0.5];
    
    SpinRate = 100 .* ones(4,1);
    EffRadius = 0.19 .* ones(4,1);
    
    [SlipAngle, SlipRatio, TireVel] = SlipEstimation( ...
        LongVel, LatVel, YawVel, TirePos, Steer, SpinRate, EffRadius);

    fprintf('Executing SlipEstimation() Test Cases: \n');
    for i = 1:numel(SlipAngle)
        fprintf('   Instance %i: \n', i);
        fprintf('      alpha = %5.2f [deg] \n', SlipAngle(i));
        fprintf('      kappa = %5.2f [ ] \n', SlipRatio(i));
        fprintf('      v_c   = %5.2f [m/s] \n', TireVel(i));
    end
    
    return;
end

%% Computation
%%% Number of Evaluations
n = numel(Steer);

%%% Tire Center Velocities
TireVel = zeros(n,3);
for i = 1:n
    TireVel(i,:) = [LongVel; LatVel; 0] + cross( [0; 0; YawVel], TirePos(i,:)' );
end

%%% Slip Angle
SlipAngle = atan2d( TireVel(:,2), TireVel(:,1) ) - Steer;

%%% Slip Ratio
SlipRatio = ( SpinRate .* EffRadius ) ./ ( norm(TireVel,2) .* cosd( SlipAngle ) ) - 1;
